simulink model "feedBack_loop"  (R2020b)
settings: Solver=VariableStepAuto  StartTime=0.0  StopTime=10.0  RelTol=1e-3
libraries: dspsrcs4 x1, SimulinkForSyDe x1
settings Model: Creator=Andrea  LastModifiedBy=Andrea

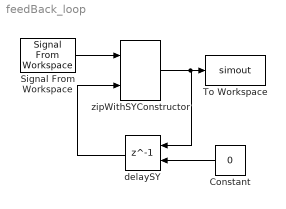
== system feedBack_loop ==
  Constant : Constant  Value=0
  Signal From Workspace : dspsrcs4/Signal From Workspace  X=s1  Ts=1  nsamps=1  OutputAfterFinalValue=Setting to zero  ignoreOrWarnInputAndFrameLengths=off  OutputFrames=off
  To Workspace : ToWorkspace  VariableName=simout  SampleTime=-1
  delaySY : Delay  DelayLength=1  InitialConditionSource=Input port
      settings: InputPortMap=u0,p4
  zipWithSYConstructor : SimulinkForSyDe/zipWithSYConstructor  SystemSampleTime=-1  VariantActivationTime=update diagram  Latency=0  AutoFrameSizeCalculation=off
      settings: SourceProductName=Simulink ForSyDe
  wires:
  zipWithSYConstructor/1 -> delaySY/1, To Workspace/1
  Signal From Workspace/1 -> zipWithSYConstructor/1
  delaySY/1 -> zipWithSYConstructor/2
  Constant/1 -> delaySY/2
